simulink model "DAB"  (R2024a)
settings: Solver=ode23tb  StartTime=0.0  StopTime=0.05  MaxStep=1e-3  RelTol=1e-3  EnableMultiTasking=on
PreLoadFcn:
  | DualActiveBridgeConverterData
undefined symbols (not defined in the file): C_HV, C_LV, Fsw, L_Inductor, Lm_Tr, Lprim_Tr, Lsec_Tr, N_Tr, Pnom, R_DCsrc1, R_DCsrc2, R_Inductor, RC_HV, RC_LV, Rm_Tr, Rprim_Tr, Rsec_Tr, Ts_Power, Vnom_HV, Vnom_LV
libraries: spsMosfetLib x8, spsSeriesRLCBranchLib x5, spsCurrentMeasurementLib x4, spsVoltageMeasurementLib x4, simulink x2, spsDCVoltageSourceLib x2, spsMeanLib x2, spsStairGeneratorLib x1, slpidlib x1, spsSawtoothGeneratorLib x1, spsLinearTransformerLib x1, spspowerguiLib x1
settings Model: SimulationMode=accelerator  Creator=The MathWorks, Inc.  LastModifiedBy=User
settings SolverCC: AlgebraicLoopSolver=TrustRegion
settings DataIOCC: LimitDataPoints=on  SaveFormat=Array  SaveOutput=off  DSMLogging=off  SaveTime=off  ReturnWorkspaceOutputs=off
settings OptimizationCC: LifeSpan=inf
settings DebuggingCC: SaveWithParameterizedLinksMsg=none  UnderspecifiedInitializationDetection=Classic  MergeDetectMultiDrivingBlocksExec=none  SolverPrmCheckMsg=warning  FcnCallInpInsideContextMsg=warning  UnconnectedInputMsg=warning  UnconnectedOutputMsg=warning  UnconnectedLineMsg=warning  StateNameClashWarn=warning  SubsystemReferenceDiagnosticForUnitTest=warning  SFUnexpectedBacktrackingDiag=warning  SFNoUnconditionalDefaultTransitionDiag=warning  SFExecutionAtInitializationDiag=none  ArithmeticOperatorsInVariantConditions=warning
settings HardwareCC: ProdBitPerPointer=32  ProdBitPerSizeT=32  ProdBitPerPtrDiffT=32  ProdLargestAtomicFloat=None  ProdIntDivRoundTo=Undefined  ProdEndianess=Unspecified  ProdWordSize=32  ProdHWDeviceType=32-bit Generic  TargetHWDeviceType=32-bit Generic
settings ModelReferenceCC: EnableRefExpFcnMdlSchedulingChecks=on  PropagateSignalLabelsOutOfModel=off
settings SFSimCC: SimUseLocalCustomCode=off  CustomCodeUndefinedFunction=UseInterfaceOnly
settings RTWCC: RTWUseLocalCustomCode=off  GPUComputeCapability=3.5  DLArmComputeVersion=19.05
settings CodeAppCC: StateflowObjectComments=on
settings GRTTargetCC: TargetFcnLib=ansi_tfl_tmw.mat  TargetLangStandard=C89/C90 (ANSI)  CombineOutputUpdateFcns=off  GRTInterface=on
settings ConfigComp: CovMetricSettings=dw  CovSaveCumulativeToWorkspaceVar=on  CovSaveSingleToWorkspaceVar=on  CovExternalEMLEnable=off  CovSFcnEnable=off

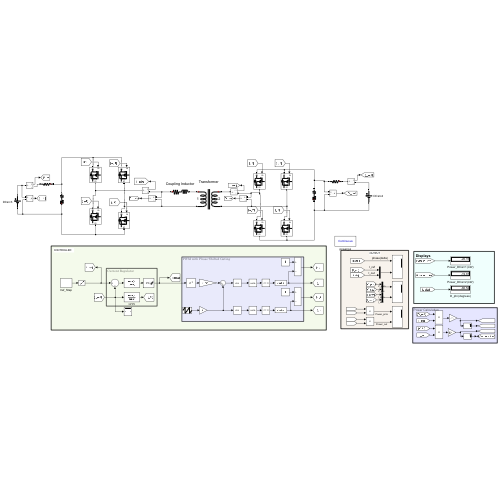
[thumbnail: Simulink's stored preview of the top-level diagram]
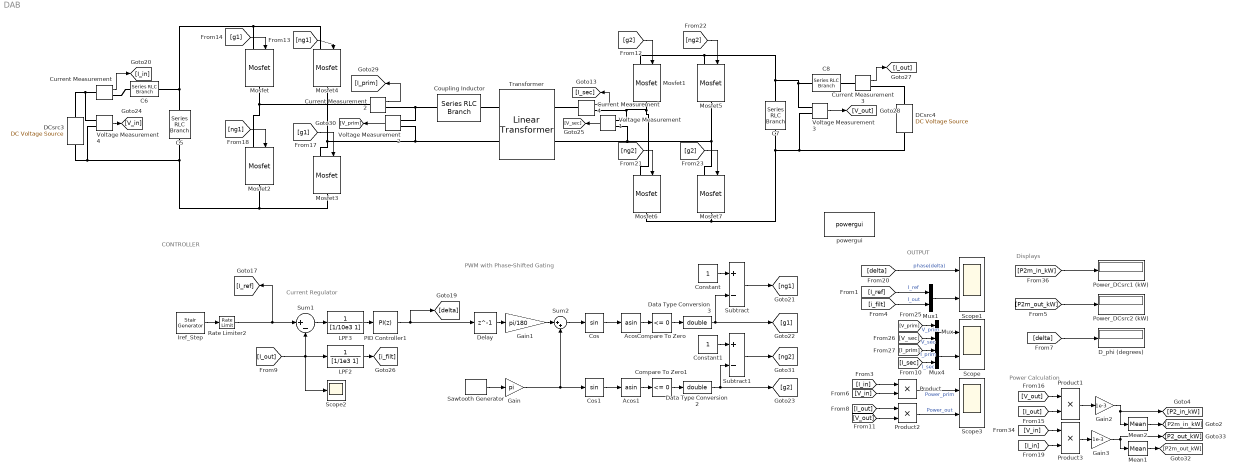
== system DAB ==
  note: Power Calculation
  note: CONTROLLER
  note: OUTPUT
  note: Displays
  note: Current Regulator
  note: PWM with Phase-Shifted Gating
  Acos : Trigonometry  Operator=asin
  Acos1 : Trigonometry  Operator=asin
  C5 : spsSeriesRLCBranchLib/Series RLC Branch  LConnTagsString=__new0  RConnTagsString=__new0  BranchType=RC  Resistance=RC_HV  Inductance=1  SetiL0=off  InitialCurrent=0  Capacitance=C_HV  Setx0=off  InitialVoltage=0  Measurements=None
  C6 : spsSeriesRLCBranchLib/Series RLC Branch  LConnTagsString=__new0  RConnTagsString=__new0  BranchType=R  Resistance=R_DCsrc1  Inductance=1  SetiL0=off  InitialCurrent=0  Capacitance=1  Setx0=off  InitialVoltage=0  Measurements=None
  C7 : spsSeriesRLCBranchLib/Series RLC Branch  LConnTagsString=__new0  RConnTagsString=__new0  BranchType=RC  Resistance=RC_LV  Inductance=1  SetiL0=off  InitialCurrent=0  Capacitance=C_LV  Setx0=off  InitialVoltage=0  Measurements=None
  C8 : spsSeriesRLCBranchLib/Series RLC Branch  LConnTagsString=__new0  RConnTagsString=__new0  BranchType=R  Resistance=R_DCsrc2  Inductance=100e-6  SetiL0=off  InitialCurrent=0  Capacitance=1  Setx0=off  InitialVoltage=0  Measurements=None
  Compare To Zero : simulink/Logic and Bit Operations/Compare To Zero  relop=<=  OutDataTypeStr=boolean
  Compare To Zero1 : simulink/Logic and Bit Operations/Compare To Zero  relop=<=  OutDataTypeStr=boolean
  Constant : Constant
  Constant1 : Constant
  Cos : Trigonometry
  Cos1 : Trigonometry
  Coupling Inductor : spsSeriesRLCBranchLib/Series RLC Branch  LConnTagsString=__new0  RConnTagsString=__new0  BranchType=RL  Resistance=R_Inductor  Inductance=L_Inductor  SetiL0=off  InitialCurrent=0  Capacitance=1e-6  Setx0=off  InitialVoltage=0  Measurements=None
  Current Measurement{,2..4} (4 alike) : spsCurrentMeasurementLib/Current Measurement  PhasorSimulation=off  OutputType=Complex  PSBequivalent=0
  DCsrc3 : spsDCVoltageSourceLib/DC Voltage Source  Amplitude=Vnom_HV  Measurements=None
  DCsrc4 : spsDCVoltageSourceLib/DC Voltage Source  Amplitude=Vnom_LV  Measurements=None
  D_phi (degrees) : Display
      settings: Format=bank  Decimation=100
  Data Type Conversion2 : DataTypeConversion  OutDataTypeStr=double  SaturateOnIntegerOverflow=off  RndMeth=Floor
  Data Type Conversion3 : DataTypeConversion  OutDataTypeStr=double  SaturateOnIntegerOverflow=off  RndMeth=Floor
  Delay : Delay  DelayLength=1  SampleTime=1/Fsw
  Gain : Gain  Gain=pi
  Gain1 : Gain  Gain=pi/180
  Gain2 : Gain  Gain=1e-3
  Gain3 : Gain  Gain=1e-3
  Iref_Step : spsStairGeneratorLib/Stair Generator  t=[0, 0.01]  e=[45, -45]  Ts=0
  LPF2 : TransferFcn  Denominator=[1/1e3 1]
  LPF3 : TransferFcn  Denominator=[1/10e3 1]
  Mean1 : spsMeanLib/Mean  Freq=Fsw  Vinit=0  Ts=0
  Mean2 : spsMeanLib/Mean  Freq=Fsw  Vinit=0  Ts=0
  Mosfet{,1..7} (8 alike) : spsMosfetLib/Mosfet  Ron=Ron_FET  Lon=0  Rd=Ron_Diode  Vfd=Vf_Diode  IC=0  Rs=Rs_FET  Cs=Cs_FET  Measurements=off
  Mux : Mux  Inputs=2
  Mux1 : Mux  Inputs=2
  Mux4 : Mux  Inputs=2
  PID Controller1 : slpidlib/PID Controller  Controller=PI  Form=Parallel  TimeDomain=Discrete-time  UseExternalTs=off  SampleTime=-1  IntegratorMethod=Forward Euler  FilterMethod=Forward Euler  ControllerParametersSource=internal  P=0.5  I=15000  UseKiTs=off  D=0  UseExternalDerivativeSource=off  N=100  UseFilter=on  TunerSelectOption=Transfer Function Based (PID Tuner App)  InitialConditionSource=internal  InitialConditionForIntegrator=0  InitialConditionForFilter=0  DifferentiatorICPrevScaledInput=0  ExternalReset=none  TrackingMode=off  Kt=1  LimitOutput=on  SatLimitsSource=internal  UpperSaturationLimit=90  LowerSaturationLimit=-90  LinearizeAsGain=on  AntiWindupMode=clamping  Kb=1  LimitIntegrator=off  UpperIntegratorSaturationLimit=inf  LowerIntegratorSaturationLimit=-inf  POutMin=[]  POutMax=[]  IOutMin=[]  IOutMax=[]  DOutMin=[]  DOutMax=[]  NOutMin=[]  NOutMax=[]  SumOutMin=[]  SumOutMax=[]  SaturationOutMin=[]  SaturationOutMax=[]  PParamMin=[]  PParamMax=[]  IParamMin=[]  IParamMax=[]  DParamMin=[]  DParamMax=[]  NParamMin=[]  NParamMax=[]  KbParamMin=[]  KbParamMax=[]  KtParamMin=[]  KtParamMax=[]  KbOutMin=[]  KbOutMax=[]  KtOutMin=[]  KtOutMax=[]  IntegratorOutMin=[]  IntegratorOutMax=[]  FilterOutMin=[]  FilterOutMax=[]  SumI1OutMin=[]  SumI1OutMax=[]  SumI2OutMin=[]  SumI2OutMax=[]  SumI3OutMin=[]  SumI3OutMax=[]  SumI4OutMin=[]  SumI4OutMax=[]  SumDOutMin=[]  SumDOutMax=[]  DifferentiatorOutMin=[]  DifferentiatorOutMax=[]  FilterDiffOutCoefMin=[]  FilterDiffOutCoefMax=[]  ReciprocalOutMin=[]  ReciprocalOutMax=[]  SumDenOutMin=[]  SumDenOutMax=[]  SumNumOutMin=[]  SumNumOutMax=[]  DivideOutMin=[]  DivideOutMax=[]  UdiffTsProdOutMin=[]  UdiffTsProdOutMax=[]  NTsProdOutMin=[]  NTsProdOutMax=[]  UintegralTsProdOutMin=[]  UintegralTsProdOutMax=[]  UngainTsProdOutMin=[]  UngainTsProdOutMax=[]  ClampingZeroOutDataTypeStr=Inherit: Inherit via back propagation  ClampingZeroOutMin=[]  ClampingZeroOutMax=[]  FilterDenConstantOutDataTypeStr=Inherit: Inherit via back propagation  FilterDenConstantOutMin=[]  FilterDenConstantOutMax=[]  PCopyOutDataTypeStr=Inherit: Inherit via back propagation  PCopyOutMin=[]  PCopyOutMax=[]  NCopyOutDataTypeStr=Inherit: Inherit via back propagation  NCopyOutMin=[]  NCopyOutMax=[]  IntegratorContinuousStateAttributes=''  IntegratorStateMustResolveToSignalObject=off  IntegratorRTWStateStorageClass=Auto  FilterContinuousStateAttributes=''  FilterStateMustResolveToSignalObject=off  FilterRTWStateStorageClass=Auto  ParallelPVariant=InternalParameters  IdealPVariant=Disabled  IVariant=InternalParameters  DVariant=Disabled  IntegratorVariant=Discrete  SatVariant=Enabled  AWVariant=DiscClampingParallel  PCopyVariant=Disabled  TRVariant=Disabled  FdbkBlocksVariant=Forward  IdealPFdbkVariant=Disabled  SatFdbkVariant=Disabled  DerivativeFilterVariant=Disabled  NVariant=Disabled  NCopyVariant=Disabled_SignalSpec  FilterICVariant=Disabled  IntegratorICVariant=InternalICs  ExternalResetVariant=Disabled  TRSumVariant=Passthrough  SumFdbkVariant=Disabled  SumVariant=Sum_PI  TsampFilterVariant=InternalTs  TsampNgainVariant=Passthrough  TsampIntegralVariant=Disabled_SignalSpec  ExternalSaturationOutDataTypeStr=Inherit: Same as second input  DerivativeSourceVariant=Disabled
  Power_DCsrc1 (kW) : Display
      settings: Format=bank  Decimation=100
  Power_DCsrc2 (kW) : Display
      settings: Format=bank  Decimation=100
  Product{,1..3} (4 alike) : Product
  Rate Limiter2 : RateLimiter  RisingSlewLimit=3000  FallingSlewLimit=-3000  SampleTimeMode=inherited
  Sawtooth Generator : spsSawtoothGeneratorLib/Sawtooth Generator  Freq=Fsw  Phase=180  Ts=0
  Scope : Scope  NumInputPorts=2
  Scope1 : Scope  NumInputPorts=2
  Scope2 : Scope
  Scope3 : Scope  NumInputPorts=2
  Subtract : Sum  Inputs=+-
  Subtract1 : Sum  Inputs=+-
  Sum1 : Sum  Inputs=|+-
  Sum2 : Sum  Inputs=|++
  Transformer : spsLinearTransformerLib/Linear Transformer  UNITS=SI  NominalPower="[ Pnom,  Fsw]"  winding1="[ Vnom_HV,  Rprim_Tr, Lprim_Tr]"  winding2="[ Vnom_HV/N_Tr,  Rsec_Tr, Lsec_Tr]"  ThreeWindings=off  winding3=[3.15e+05 0.7938 0.084225]  RmLm="[ Rm_Tr,  Lm_Tr]"  Measurements=None  DataType=on
  Voltage Measurement{1..4} (4 alike) : spsVoltageMeasurementLib/Voltage Measurement  PhasorSimulation=off  OutputType=Complex  PSBequivalent=0
  powergui : spspowerguiLib/powergui  Priority=1  SimulationMode=Continuous  SampleTime=Ts_Power  frequency=60  Iterations=50  frequencyindice=0  Pbase=100e6  ErrMax=1e-4  UnitsV=kV  UnitsW=MW  buscounter=0  FunctionMessages=off  echomessages=off  EnableUseOfTLC=off  CurrentSourceSwitches=on  DisableSnubberDevices=off  DisableRonSwitches=off  DisableVfSwitches=off  DisplayEquations=off  AutomaticDiscreteSolvers=off  SolverType=Tustin/Backward Euler (TBE)  Interpol=off  ExternalGateDelay=off  methode=off  Ts=10  x0status=blocks  SPID=on  SwTol=0  HookPort=off  NonlinearTolerance=1e-4  nMaxIteration=100  ContinueOnMaxIteration=off  RestoreLinks=warning  ResistiveCurrentMeasurement=off  Frange=[0:2:500]  Ylog=off  Xlog=on  ShowGrid=off  save=off  variable=ZData  structure=0  ZoomFFT=off  StartTime=0.0  cycles=1  DisplayStyle=1  fundamental=60  FreqAxis=off  MaxFrequency=1000  frequencyindicesteady=1  RmsSteady=1  display=off
  wires:
  [I_out] -> Product1/2
  [V_out] -> Product1/1
  Product1/1 -> Gain2/1
  Gain2/1 -> Mean2/1, [P2_in_kW]
  [delta] -> Scope1/1  "phase(delta)"
  [I_ref] -> Mux1/1  "I_ref"
  [i_filt] -> Mux1/2  "I_out"
  Rate Limiter2/1 -> [I_ref], Sum1/1
  Iref_Step/1 -> Rate Limiter2/1
  Mean2/1 -> [P2m_in_kW]
  [P2m_out_kW] -> Power_DCsrc2 (kW)/1
  [delta] -> D_phi (degrees)/1
  Voltage Measurement2/1 -> [V_prim]
  [ng2] -> Mosfet5/1
  [g1] -> Mosfet/1
  [g2] -> Mosfet1/1
  [g2] -> Mosfet7/1
  [ng1] -> Mosfet2/1
  Current Measurement3/1 -> [I_out]
  Voltage Measurement1/1 -> [V_sec]
  Voltage Measurement3/1 -> [V_out]
  [g1] -> Mosfet3/1
  Current Measurement2/1 -> [I_prim]
  [ng1] -> Mosfet4/1
  [ng2] -> Mosfet6/1
  Gain/1 -> Cos1/1, Sum2/2
  Gain1/1 -> Sum2/1
  Acos1/1 -> Compare To Zero1/1
  Cos1/1 -> Acos1/1
  Compare To Zero/1 -> Data Type Conversion3/1
  Data Type Conversion3/1 -> Subtract/2, [g1]
  LPF3/1 -> PID Controller1/1
  [I_out] -> Sum1/2, Scope2/1, LPF2/1
  PID Controller1/1 -> Delay/1, [delta]
  Sum1/1 -> LPF3/1
  Constant1/1 -> Subtract1/1
  Constant/1 -> Subtract/1
  Data Type Conversion2/1 -> Subtract1/2, [g2]
  Sum2/1 -> Cos/1
  Cos/1 -> Acos/1
  Subtract/1 -> [ng1]
  Sawtooth Generator/1 -> Gain/1
  Acos/1 -> Compare To Zero/1
  LPF2/1 -> [i_filt]
  Compare To Zero1/1 -> Data Type Conversion2/1
  Subtract1/1 -> [ng2]
  Delay/1 -> Gain1/1
  Mux1/1 -> Scope1/2
  [I_in] -> Product/1
  [V_in] -> Product/2
  [V_out] -> Product2/2
  [I_out] -> Product2/1
  Product/1 -> Scope3/1  "Power_prim"
  Product2/1 -> Scope3/2  "Power_out"
  Current Measurement4/1 -> [I_sec]
  [V_prim] -> Mux/1  "V_prim"
  Mux/1 -> Scope/1
  [V_sec] -> Mux/2  "V_sec"
  [I_prim] -> Mux4/1  "I_prim"
  [I_sec] -> Mux4/2  "I_sec"
  Mux4/1 -> Scope/2
  Current Measurement/1 -> [I_in]
  Voltage Measurement4/1 -> [V_in]
  [I_in] -> Product3/2
  Gain3/1 -> Mean1/1, [P2_out_kW]
  Mean1/1 -> [P2m_out_kW]
  Product3/1 -> Gain3/1
  [V_in] -> Product3/1
  [P2m_in_kW] -> Power_DCsrc1 (kW)/1
  connections:
  Voltage Measurement2/LConn1 -- Current Measurement2/RConn1 -- Coupling Inductor/LConn1
  C5/LConn1 -- Mosfet3/RConn1 -- Mosfet2/RConn1 -- Voltage Measurement4/LConn2 -- DCsrc3/LConn1
  C7/RConn1 -- Mosfet1/LConn1 -- Mosfet5/LConn1 -- C8/RConn1 -- Voltage Measurement3/LConn1
  Mosfet2/LConn1 -- Current Measurement2/LConn1 -- Mosfet/RConn1
  Transformer/LConn1 -- Coupling Inductor/RConn1
  C5/RConn1 -- Mosfet/LConn1 -- Mosfet4/LConn1 -- C6/LConn1
  Mosfet6/LConn1 -- Mosfet1/RConn1 -- Current Measurement4/RConn1 -- Voltage Measurement1/LConn1
  C7/LConn1 -- Mosfet7/RConn1 -- Mosfet6/RConn1 -- Voltage Measurement3/LConn2 -- DCsrc4/LConn1
  Mosfet4/RConn1 -- Voltage Measurement2/LConn2 -- Transformer/LConn2 -- Mosfet3/LConn1
  Transformer/RConn2 -- Voltage Measurement1/LConn2 -- Mosfet5/RConn1 -- Mosfet7/LConn1
  Current Measurement4/LConn1 -- Transformer/RConn1
  Current Measurement/LConn1 -- Voltage Measurement4/LConn1 -- DCsrc3/RConn1
  Current Measurement/RConn1 -- C6/RConn1
  Current Measurement3/LConn1 -- C8/LConn1
  Current Measurement3/RConn1 -- DCsrc4/RConn1
